simulink model "sl_drivepose"  (Simulink 7.7)
settings: Solver=ode45  StartTime=0.0  StopTime=20.0  MaxStep=0.05  RelTol=1e-3
undefined symbols (not defined in the file or in its folder): xg
libraries: roblocks x1, simulink x1
settings Model: Creator=pic  LastModifiedBy=corkep
settings DataIOCC: LimitDataPoints=off  SaveState=on  ReturnWorkspaceOutputs=on
settings DebuggingCC: StrictBusMsg=Warning

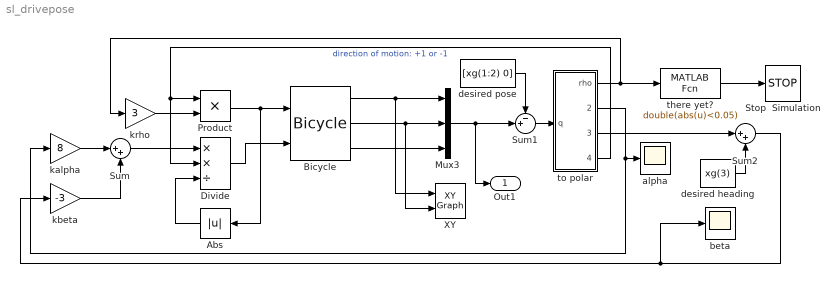
== system sl_drivepose ==
  Abs : Abs
  Bicycle : roblocks/Dynamics/Bicycle  SystemSampleTime=-1  accel=1  vlim=1  alim=1  L=1  x0=x0  handbrake=0
  Divide : Product  Inputs=**/
  Mux3 : Mux  Inputs=3
  Product : Product  RndMeth=Zero
  Stop  Simulation : Stop
  Sum : Sum  Inputs=|++
  Sum1 : Sum  Inputs=-+|
  Sum2 : Sum  Inputs=|++
  XY : simulink/Sinks/XY Graph  SystemSampleTime=-1  xmin=0  xmax=10  ymin=0  ymax=10  st=-1
  alpha : Scope
  beta : Scope
      settings: SaveName=ScopeData2
  desired heading : Constant  Value=xg(3)
  desired pose : Constant  Value=[xg(1:2) 0]
  kalpha : Gain  Gain=8
  kbeta : Gain  Gain=-3
  krho : Gain  Gain=3
  there yet? : MATLABFcn  MATLABFcn=double(abs(u)<0.05)  OutputSignalType=real
  to polar : Subsystem
  Out1 : Outport
  wires:
  Mux3/1 -> Out1/1, Sum1/2
  Bicycle/1 -> Mux3/1, XY/1
  Bicycle/2 -> Mux3/2, XY/2
  Bicycle/3 -> Mux3/3
  to polar/2(alpha) -> kalpha/1, alpha/1
  kalpha/1 -> Sum/1
  kbeta/1 -> Sum/2
  Product/1 -> Bicycle/1, Abs/1
  krho/1 -> Product/2
  to polar/1(rho) -> there yet?/1, krho/1
  to polar/4(direction) -> Product/1, Divide/2  "direction of motion: +1 or -1"
  desired pose/1 -> Sum1/1
  Sum1/1 -> to polar/1(q)
  Sum/1 -> Divide/1
  there yet?/1 -> Stop  Simulation/1
  to polar/3(beta) -> Sum2/1
  Sum2/1 -> kbeta/1, beta/1
  desired heading/1 -> Sum2/2
  Divide/1 -> Bicycle/2
  Abs/1 -> Divide/3

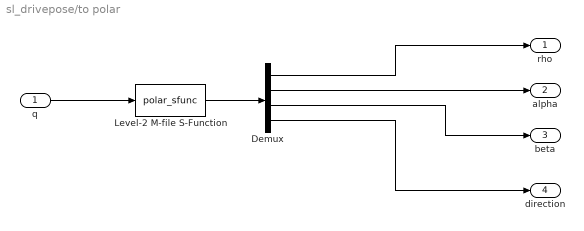
== system sl_drivepose/to polar ==
  q : Inport
  Demux : Demux
  Level-2 M-file S-Function : M-S-Function  FunctionName=polar_sfunc
  rho : Outport
  alpha : Outport  Port=2
  beta : Outport  Port=3
  direction : Outport  Port=4
  wires:
  Demux/3 -> beta/1
  q/1 -> Level-2 M-file S-Function/1
  Level-2 M-file S-Function/1 -> Demux/1
  Demux/1 -> rho/1
  Demux/2 -> alpha/1
  Demux/4 -> direction/1
